simulink model "SatSIM_revJuli16_07"  (R2015a)
settings: Solver=ode15s  StartTime=0.0  StopTime=15000  RelTol=1e-3
values from neighbouring files (symbols this model uses):
  dfy = d    [dfy.m]
  s = sin(ir)    [B_dipole_June16_2.m]    (also in LTC_to_NED.m = sin(e); LTC_to_NED_edit.m = sin(e); TimeConverter.m = fix(sec); read_epoch.m = ((e-h)*60)-min)
undefined symbols (not defined in the file or in its folder): B_dipole_June16_2, DCM_ROI, deg, Earth_MagField_may16_Rev4, InertiaMoment3, LTC_to_NED_edit, rad, read_epochS, sec_to_ymdhms2, SimpleB5
libraries: aerolibconvert2 x13, aerolibutil x7, aerolibtransform2 x4, dspmtrx3 x3, vrlib x2, aerolibanim x1
(part 2 of 2)

== matlab function SatSIM_revJuli16_07/Environtments/Transformation Coordinate/ECEF to alt,lat,long/  ==
  data: lat input; latitude output
function latitude= fcn(lat)
%#codegen
%jika sudut lebih besar dari 90 derajat maka
a=(abs(lat))/360;
if a<1
    latitude=abs(lat);
else
    b=fix(a);
    latitude=abs(lat-(b*360));
end
end

== matlab function SatSIM_revJuli16_07/Environtments/Transformation Coordinate/ECEF to alt,lat,long/    ==
  data: long input; longitude output
function longitude= fcn(long)
%#codegen
%jika sudut lebih besar dari 360 derajat maka
%untuk sudut <360, sudut=sudut
%untuk sudut >360
a=(abs(long))/360;
if a<1
    longitude=abs(long);
else
    b=fix(a);
    longitude=abs(long-(b*360));
end
end

== matlab function SatSIM_revJuli16_07/Environtments/Transformation Coordinate/ECEF to NED/Matrix Rotation ECEF to Local Horizon ==
  data: Rlg output; long input; lat input
function Rlg = RLG(long,lat)
%#codegen
%alt = Altitude
%long = Longitude
%Lat = Latitude

%Matrix rotation from ECEF to Local Horizon
R1=[-sind(lat)*cosd(long) -sind(lat)*sind(long) cosd(lat);...
    -sind(long) cosd(long) 0;...
    -cosd(lat)*cosd(long) -cosd(lat)*sind(long) -sind(lat)];

Rlg = R1;

== matlab function SatSIM_revJuli16_07/Environtments/Transformation Coordinate/ECEF to alt,lat,long/alt,long,lat ==
  data: xG input; alt output; yG input; zG input; long output; lat output
function [alt, long, lat] = XYZtoALL(xG,yG,zG)
%#codegen
%alttitude
alt=((xG^2)+(yG^2)+(zG^2))^0.5;

%longitude
long=atand(yG/xG);

%latitude
lat=atand(zG/(((xG^2)+(yG^2))^0.5));

end

== matlab function SatSIM_revJuli16_07/OUTPUT/date/s2hms ==
  data: secs input; hour output; min output; sec output
function [hour,min,sec]=s2hms(secs)
%S2HMS converts seconds to integer hour,minute,seconds
%
sec=round(secs);

h=fix(sec/3600);
if h<24
    hour=floor(sec/3600);
else
    a=fix((sec/3600)/24);
    hour=floor((sec/3600)-(24*a));
end

min=floor(rem(sec,3600)/60);
sec=round(rem(sec,60));
end

== matlab function SatSIM_revJuli16_07/Actuator/currents Y ==
  data: Imax input; Ib output; Iy input
function Ib = currents(Imax,Iy)
%#Currents filter
if Iy>(-1*Imax) && Iy<Imax
    Ib=Iy;
else
    if Iy>0 %positif
        Ib=Imax;
    else % negatif
        Ib=-1*Imax;
    end
end
end

== matlab function SatSIM_revJuli16_07/Actuator/currents Z ==
  data: Imax input; Ic output; Iz input
function Ic = currents(Imax,Iz)
%#Currents filter
if Iz>(-1*Imax) && Iz<Imax
    Ic=Iz;
else
    if Iz>0 %positif
        Ic=Imax;
    else % negatif
        Ic=-1*Imax;
    end
end
end

== matlab function SatSIM_revJuli16_07/dynamic inertial/w(t) to Quaternion/quaternion derivative ==
  data: q0 input; q1 input; q2 input; q3 input; qdot output
function qdot   = q( q0,q1,q2,q3 )
%CONVERTION FROM ANGULAR VELOCITY TO QUATERNION
%-------------------------------------------------------------------------%
%   this block need and looping input and output so maybe there have a
%   singularities
%   OMG=angular velociti
%   with componen = [w1 w2 w3];
%   unit in degree/s
%   q have dimention 1x4, q=[q0 q1 q2 q3], q4=q0
%-------------------------------------------------------------------------%
%lets divine a matrix with dimention 4x3
qdot=[q0 -q3 q2;...
    q3 q0 -q1;...
    -q2 q1 q0;...
    -q1 -q2 -q3];
%--------------------------------END---------------------------------------%
end
